simulink model "SIM_CSTR"  (R2023b)
settings: Solver=VariableStepAuto  StartTime=0.0  StopTime=30  RelTol=1e-3
values from neighbouring files (symbols this model uses):
  Ts = 0.05    [NMPC_CSTR.m]
  u0 = 300    [NMPC_CSTR.m]
libraries: mpclib x1, simulink x1, SignalEditorBlockLib x1
settings Model: Creator=akeebismail  LastModifiedBy=akeebismail

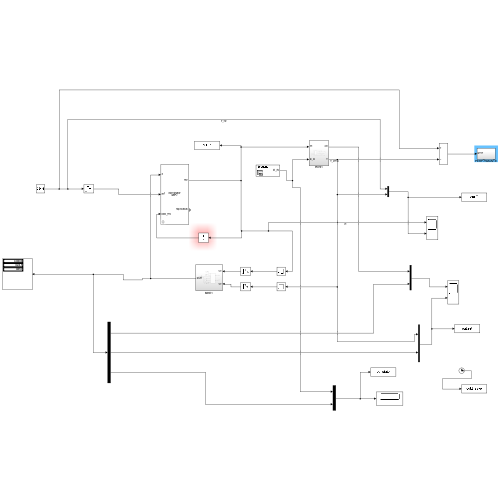
[thumbnail: Simulink's stored preview of the top-level diagram]
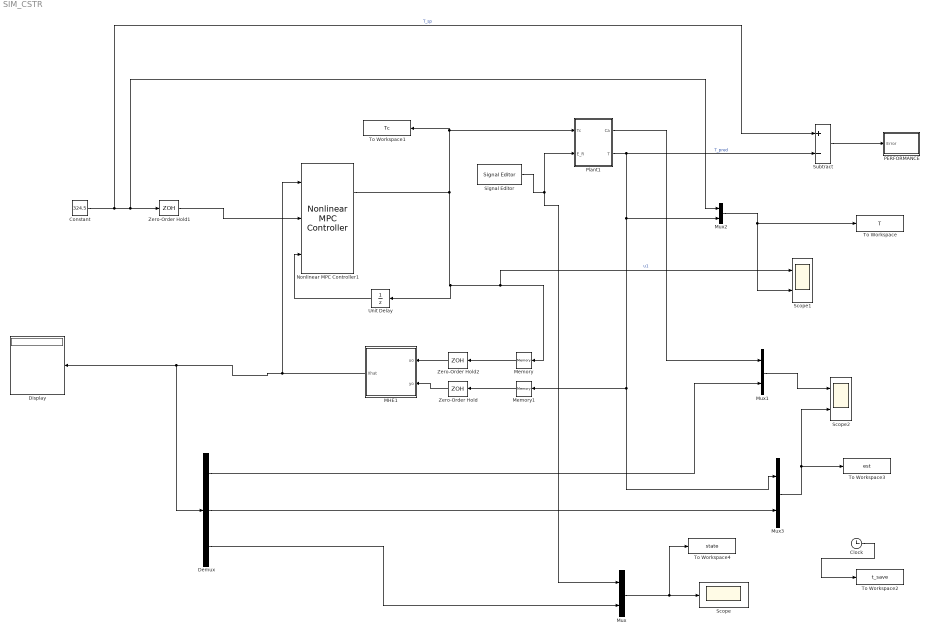
== system SIM_CSTR ==
  Clock : Clock
  Constant : Constant  Value=324.5
  Demux : Demux  Outputs=3
  Display : Display
  MHE1 : Subsystem
  Memory : Memory  InitialCondition=300
  Memory1 : Memory  InitialCondition=324.5
  Mux{,1..3} (4 alike) : Mux  Inputs=2
  Nonlinear MPC Controller1 : mpclib/Nonlinear MPC Controller  nlmpcobj=nlobj  UseObjectTs=on  UseMEX=off  md_enabled=off  mvtarget_enabled=off  param_enabled=off  cost_enabled=off  mvseq_enabled=off  stateseq_enabled=off  ovseq_enabled=off  slack_enabled=off  status_enabled=on  ov_min=off  ov_max=off  mv_min=off  mv_max=off  mvrate_min=off  mvrate_max=off  state_min=off  state_max=off  ov_weight=off  mv_weight=off  mvrate_weight=off  ecr_weight=off  nlp_initialize=off
  PERFORMANCE : Subsystem
  Plant1 : Subsystem
  Scope : Scope
  Scope1 : Scope  NumInputPorts=2
  Scope2 : Scope  NumInputPorts=2
  Signal Editor : SignalEditorBlockLib/Signal Editor  FileName=E_R.mat  ActiveScenario=Scenario  ActiveSignal=E_R  IsBus=off  OutputBusObjectStr=Bus: BusObject  SampleTime=Ts  Interpolate=off  ZeroCross=off  OutputAfterFinalValue=Setting to zero  Unit=inherit  PreserveSignalName=on  ApplySigPropsToAllScenarios=on  ApplySigPropsToAllSignals=off
  Subtract : Sum  Inputs=+-
  To Workspace : ToWorkspace  VariableName=T  SaveFormat=Timeseries  SampleTime=Ts
  To Workspace1 : ToWorkspace  VariableName=Tc  SaveFormat=Timeseries  SampleTime=Ts
  To Workspace2 : ToWorkspace  VariableName=t_save  SaveFormat=Timeseries  SampleTime=Ts
  To Workspace3 : ToWorkspace  VariableName=est  SaveFormat=Timeseries  SampleTime=Ts
  To Workspace4 : ToWorkspace  VariableName=state  SaveFormat=Timeseries  SampleTime=Ts
  Unit Delay : UnitDelay  InitialCondition=u0  SampleTime=-1  HasFrameUpgradeWarning=on
  Zero-Order Hold : ZeroOrderHold  SampleTime=Ts
  Zero-Order Hold1 : ZeroOrderHold  SampleTime=Ts
  Zero-Order Hold2 : ZeroOrderHold  SampleTime=Ts
  wires:
  Plant1/2(T) -> Mux3/1, Memory1/1, Mux2/2, Subtract/2  "T_pred"
  Mux2/1 -> To Workspace/1, Scope1/2
  Zero-Order Hold/1 -> MHE1/2(yo)
  Nonlinear MPC Controller1/1 -> To Workspace1/1, Plant1/1(Tc), Unit Delay/1, Scope1/1, Memory/1  "u1"
  Constant/1 -> Subtract/1, Mux2/1, Zero-Order Hold1/1  "T_sp"
  Zero-Order Hold1/1 -> Nonlinear MPC Controller1/2
  Unit Delay/1 -> Nonlinear MPC Controller1/3
  Memory/1 -> Zero-Order Hold2/1
  MHE1/1(Xhat) -> Nonlinear MPC Controller1/1, Demux/1, Display/1
  Mux1/1 -> Scope2/1
  Mux3/1 -> To Workspace3/1, Scope2/2
  Signal Editor/1 -> Mux/1, Plant1/2(E_R)
  Demux/3 -> Mux/2
  Demux/2 -> Mux3/2
  Demux/1 -> Mux1/2
  Plant1/1(Ca) -> Mux1/1
  Mux/1 -> To Workspace4/1, Scope/1
  Memory1/1 -> Zero-Order Hold/1
  Zero-Order Hold2/1 -> MHE1/1(uo)
  Clock/1 -> To Workspace2/1
  Subtract/1 -> PERFORMANCE/1(Error)

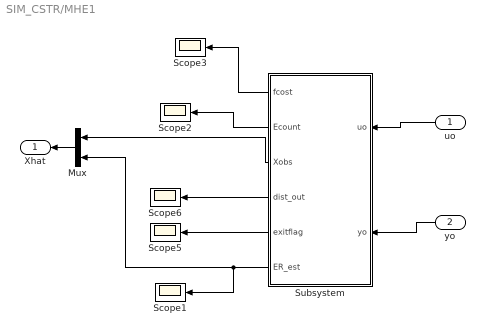
== system SIM_CSTR/MHE1 ==
  uo : Inport
  yo : Inport  Port=2
  Mux : Mux  Inputs=2
  Scope{1..3,5..6} (5 alike) : Scope
  Subsystem : Subsystem
  Xhat : Outport
  wires:
  uo/1 -> Subsystem/1(uo)
  yo/1 -> Subsystem/2(yo)
  Subsystem/1(fcost) -> Scope3/1
  Subsystem/2(Ecount) -> Scope2/1
  Subsystem/6(ER_est) -> Mux/2, Scope1/1
  Subsystem/5(exitflag) -> Scope5/1
  Subsystem/4(dist_out) -> Scope6/1
  Mux/1 -> Xhat/1
  Subsystem/3(Xobs) -> Mux/1

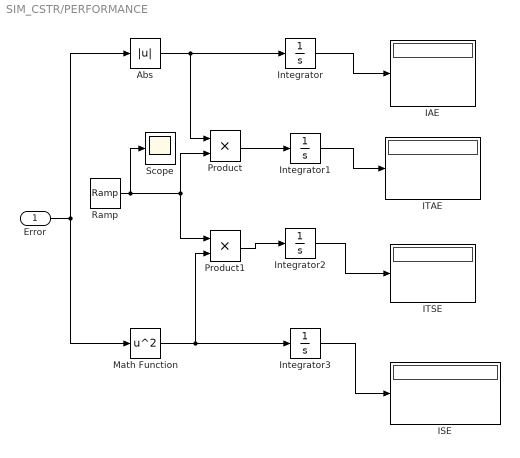
== system SIM_CSTR/PERFORMANCE ==
  Error : Inport
  Abs : Abs  SaturateOnIntegerOverflow=off
  IAE : Display
  ISE : Display
  ITAE : Display
  ITSE : Display
  Integrator{,1..3} (4 alike) : Integrator
  Math Function : Math  Operator=square  SignedPower=on
  Product : Product  RndMeth=Zero
  Product1 : Product  RndMeth=Zero
  Ramp : simulink/Sources/Ramp  slope=1  start=0  InitialOutput=0
  Scope : Scope
  wires:
  Error/1 -> Math Function/1, Abs/1
  Abs/1 -> Integrator/1, Product/1
  Integrator/1 -> IAE/1
  Ramp/1 -> Product/2, Product1/1, Scope/1
  Math Function/1 -> Integrator3/1, Product1/2
  Product1/1 -> Integrator2/1
  Product/1 -> Integrator1/1
  Integrator3/1 -> ISE/1
  Integrator2/1 -> ITSE/1
  Integrator1/1 -> ITAE/1

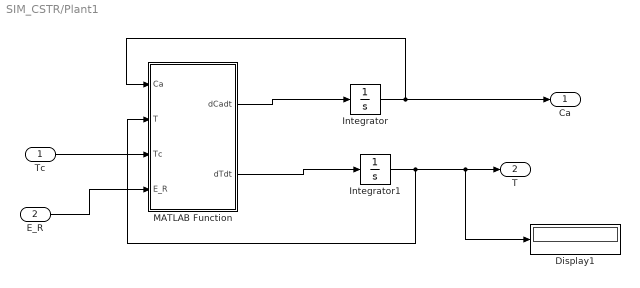
== system SIM_CSTR/Plant1 ==
  Tc : Inport
  E_R : Inport  Port=2
  Display1 : Display
  Integrator : Integrator  InitialCondition=0.877
  Integrator1 : Integrator  InitialCondition=324.5
  MATLAB Function : MATLAB Function  TreatAsAtomicUnit=on
  Ca : Outport
  T : Outport  Port=2
  wires:
  Integrator1/1 -> Display1/1, T/1, MATLAB Function/2(T)
  MATLAB Function/2(dTdt) -> Integrator1/1
  Integrator/1 -> Ca/1, MATLAB Function/1(Ca)
  MATLAB Function/1(dCadt) -> Integrator/1
  Tc/1 -> MATLAB Function/3(Tc)
  E_R/1 -> MATLAB Function/4(E_R)

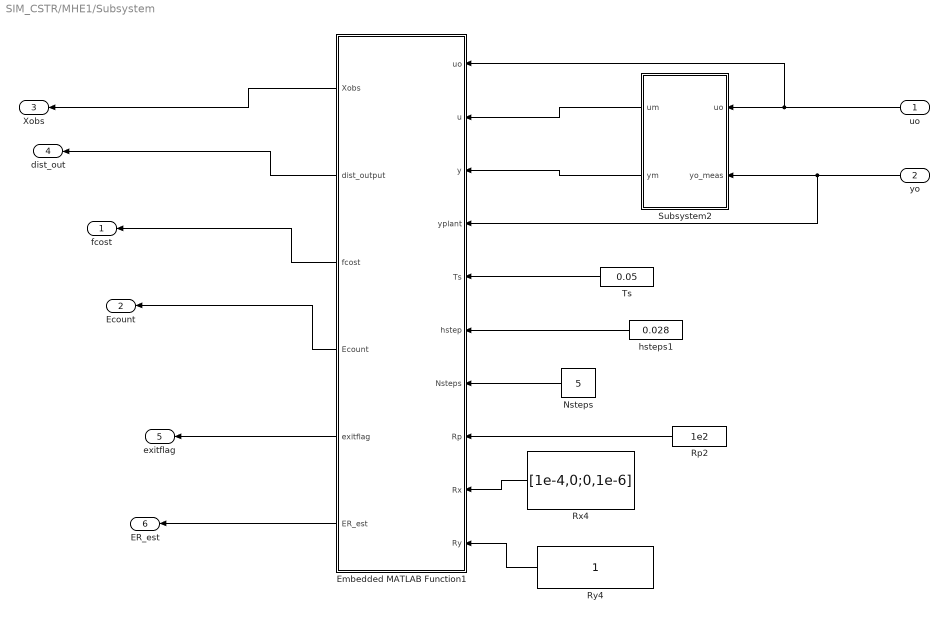
== system SIM_CSTR/MHE1/Subsystem ==
  uo : Inport
  yo : Inport  Port=2
  Embedded MATLAB Function1 : MATLAB Function  TreatAsAtomicUnit=on
  Nsteps : Constant  Value=5
  Rp2 : Constant  Value=1e2
  Rx4 : Constant  Value=[1e-4,0;0,1e-6]
  Ry4 : Constant
  Subsystem2 : Subsystem
  Ts : Constant  Value=0.05
  hsteps1 : Constant  Value=0.028
  fcost : Outport  VectorParamsAs1DForOutWhenUnconnected=off
  Ecount : Outport  Port=2  VectorParamsAs1DForOutWhenUnconnected=off
  Xobs : Outport  Port=3  VectorParamsAs1DForOutWhenUnconnected=off
  dist_out : Outport  Port=4  VectorParamsAs1DForOutWhenUnconnected=off
  exitflag : Outport  Port=5  VectorParamsAs1DForOutWhenUnconnected=off
  ER_est : Outport  Port=6  VectorParamsAs1DForOutWhenUnconnected=off
  wires:
  Subsystem2/1(um) -> Embedded MATLAB Function1/2(u)
  Subsystem2/2(ym) -> Embedded MATLAB Function1/3(y)
  yo/1 -> Embedded MATLAB Function1/4(yplant), Subsystem2/2(yo_meas)
  uo/1 -> Embedded MATLAB Function1/1(uo), Subsystem2/1(uo)
  Nsteps/1 -> Embedded MATLAB Function1/7(Nsteps)
  hsteps1/1 -> Embedded MATLAB Function1/6(hstep)
  Embedded MATLAB Function1/3(fcost) -> fcost/1
  Embedded MATLAB Function1/4(Ecount) -> Ecount/1
  Rp2/1 -> Embedded MATLAB Function1/8(Rp)
  Rx4/1 -> Embedded MATLAB Function1/9(Rx)
  Ry4/1 -> Embedded MATLAB Function1/10(Ry)
  Embedded MATLAB Function1/1(Xobs) -> Xobs/1
  Embedded MATLAB Function1/2(dist_output) -> dist_out/1
  Embedded MATLAB Function1/5(exitflag) -> exitflag/1
  Embedded MATLAB Function1/6(ER_est) -> ER_est/1
  Ts/1 -> Embedded MATLAB Function1/5(Ts)

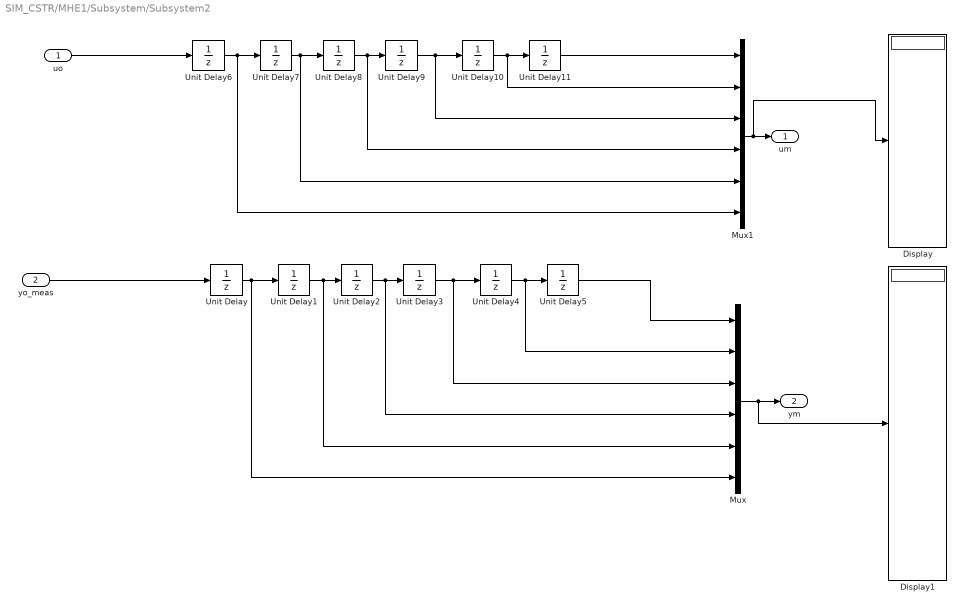
== system SIM_CSTR/MHE1/Subsystem/Subsystem2 ==
  uo : Inport
  yo_meas : Inport  Port=2
  Display : Display
  Display1 : Display
  Mux : Mux  Inputs=6
  Mux1 : Mux  Inputs=6
  Unit Delay{,1..5} (6 alike) : UnitDelay  InitialCondition=324.5  SampleTime=Ts  HasFrameUpgradeWarning=on
  Unit Delay{6..11} (6 alike) : UnitDelay  InitialCondition=300  SampleTime=Ts  HasFrameUpgradeWarning=on
  um : Outport  VectorParamsAs1DForOutWhenUnconnected=off
  ym : Outport  Port=2  VectorParamsAs1DForOutWhenUnconnected=off
  wires:
  Unit Delay/1 -> Unit Delay1/1, Mux/6
  Unit Delay1/1 -> Unit Delay2/1, Mux/5
  Unit Delay2/1 -> Unit Delay3/1, Mux/4
  Unit Delay3/1 -> Unit Delay4/1, Mux/3
  Unit Delay4/1 -> Unit Delay5/1, Mux/2
  uo/1 -> Unit Delay6/1
  Unit Delay6/1 -> Mux1/6, Unit Delay7/1
  Unit Delay7/1 -> Mux1/5, Unit Delay8/1
  Unit Delay8/1 -> Mux1/4, Unit Delay9/1
  Unit Delay9/1 -> Mux1/3, Unit Delay10/1
  Unit Delay10/1 -> Unit Delay11/1, Mux1/2
  Mux/1 -> ym/1, Display1/1
  Mux1/1 -> um/1, Display/1
  Unit Delay11/1 -> Mux1/1
  Unit Delay5/1 -> Mux/1
  yo_meas/1 -> Unit Delay/1

== matlab function SIM_CSTR/MHE1/Subsystem/Embedded MATLAB Function1 ==
  data: uo input; Xobs output size=[2,1]; dist_output output size=[1,1]; u input; y input; yplant input; Ts input; hstep input; Nsteps input; Rp input; fcost output size=[1,1]; Rx input; Ry input; Ecount output size=[1,1]; exitflag output size=[1,1]; ER_est output size=[1,1]
function [Xobs,dist_output,fcost,Ecount,exitflag,ER_est] =MHE(uo,u,y,yplant,Ts,hstep,Nsteps,Rp,Rx,Ry)

%#codegen
coder.extrinsic('MHE_compute','clear_var');

um=[u(1),u(2),u(3),u(4),u(5),u(6)] ;
 

ymeas=[y(1),y(2),y(3),y(4),y(5),y(6)] ;


    
   

% SAMPLING TIME FOR DISCRETIZATION
%hstep=1; %sampling time of 10 is with less interation while 5 is smoother but higher interaction
%Nsteps=1 ;% Nsteps=10 ; % Nsteps=20 ;


d_initial=[0.877;324.5;8750]   ;
%d_MIN_colvector =[0;0;100]  ;
d_MIN_colvector =[0.3;300;2000]  ;
d_MAX_colvector =[1.5;360;10000]  ;
%%%%%%%%%%%%%%%%%%%%%%%%%%%%%%%%%%%%%%%
%Initializing variables
fcost=inf  ;
Xobs=[0;0]  ;
%d_opt=[0;0]  ;
dist_output = [0]  ;
ER_est=[0]  ;
Ecount=0  ;
exitflag=2   ;

% [Xobs,dist_output,fcost,Ecount,exitflag]=MHE_compute(uo,um,ymeas,yplant...
%                                         ,hstep,Nsteps,Nmhe,Rp,Rx,Ry...
%                                         ,p_initial, p_MIN_colvector,p_MAX_colvector)
[Xobs,dist_output,ER_est,fcost,Ecount,exitflag]=MHE_compute(uo,um,ymeas...
                                        ,yplant,Ts,hstep,Nsteps,Rp,Rx,Ry...
                                        ,d_initial, d_MIN_colvector,d_MAX_colvector);

== matlab function SIM_CSTR/Plant1/MATLAB Function ==
  data: Ca input; dCadt output; T input; Tc input; dTdt output; E_R input
function [dCadt,dTdt] = fcn(Ca,T,Tc,E_R)

values = {100,5e4,350,100,1000,0.239,7.2e10,5e4,1};
[F,delta_H,Tf,V,rho,Cp,k0,U_A,Caf] = values{:};

% Rate constant (Arrhenius equation)
        k = k0 * exp(-E_R / T);
        
        % Mass balance for Ca
        dCadt = F/V * (Caf - Ca) - k * Ca;
        
        % Energy balance for T
        dTdt = F/V * (Tf - T) + (delta_H / (rho * Cp)) * k * Ca + (U_A / (rho * Cp * V)) * (Tc - T);


end
